simulink model "pratica8S"  (R2021b)
settings: Solver=VariableStepAuto  StartTime=0.0  StopTime=24.00  RelTol=1e-3
undefined symbols (not defined in the file): Ac, Bc, Cc, Cd, Dc, F, H, R, T0
settings Model: Creator=carlo  LastModifiedBy=carlo

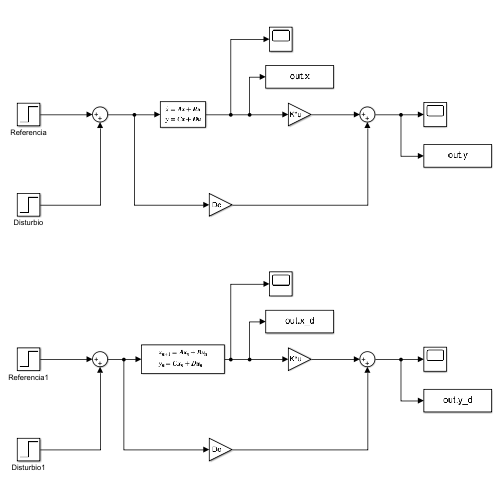
[thumbnail: Simulink's stored preview of the top-level diagram]
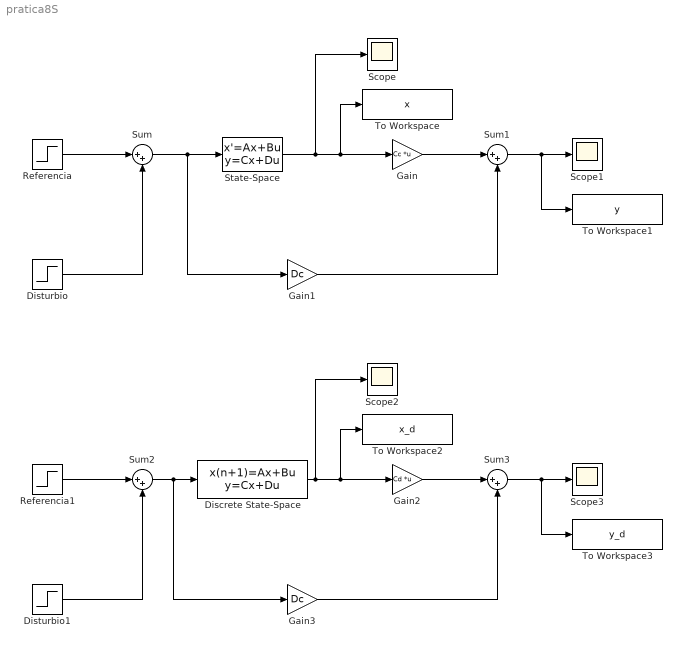
== system pratica8S ==
  Discrete State-Space : DiscreteStateSpace  A=F  B=H  C=[1 0; 0 1]  D=[0 ; 0]  SampleTime=T0
  Disturbio : Step  Time=0  After=R  SampleTime=0
  Disturbio1 : Step  Time=0  After=R  SampleTime=0
  Gain : Gain  Gain=Cc  Multiplication=Matrix(K*u)
  Gain1 : Gain  Gain=Dc
  Gain2 : Gain  Gain=Cd  Multiplication=Matrix(K*u)
  Gain3 : Gain  Gain=Dc
  Referencia : Step  Time=0  After=R  SampleTime=0
  Referencia1 : Step  Time=0  After=R  SampleTime=0
  Scope{,1..3} (4 alike) : Scope
  State-Space : StateSpace  A=Ac  B=Bc  C=[1 0; 0 1]  D=[0; 0]  InitialCondition=0
  Sum{,1..3} (4 alike) : Sum  Inputs=|++
  To Workspace : ToWorkspace  VariableName=x  SaveFormat=Timeseries  SampleTime=-1
  To Workspace1 : ToWorkspace  VariableName=y  SaveFormat=Timeseries  SampleTime=-1
  To Workspace2 : ToWorkspace  VariableName=x_d  SaveFormat=Timeseries  SampleTime=-1
  To Workspace3 : ToWorkspace  VariableName=y_d  SaveFormat=Timeseries  SampleTime=-1
  wires:
  Referencia/1 -> Sum/1
  Disturbio/1 -> Sum/2
  Sum/1 -> Gain1/1, State-Space/1
  Gain/1 -> Sum1/1
  State-Space/1 -> Scope/1, To Workspace/1, Gain/1
  Gain1/1 -> Sum1/2
  Sum1/1 -> To Workspace1/1, Scope1/1
  Disturbio1/1 -> Sum2/2
  Referencia1/1 -> Sum2/1
  Sum2/1 -> Discrete State-Space/1, Gain3/1
  Gain2/1 -> Sum3/1
  Discrete State-Space/1 -> Scope2/1, To Workspace2/1, Gain2/1
  Sum3/1 -> To Workspace3/1, Scope3/1
  Gain3/1 -> Sum3/2
